simulink model "IWP_FL_ToBeChecked"  (R2022b)
settings: Solver=FixedStepAuto  StartTime=0.0  StopTime=100  RelTol=1e-3
undefined symbols (not defined in the file): a11_num, a12_num, a21_num, a22_num, g, K_aug, mc_num
settings Model: Creator=User  LastModifiedBy=User

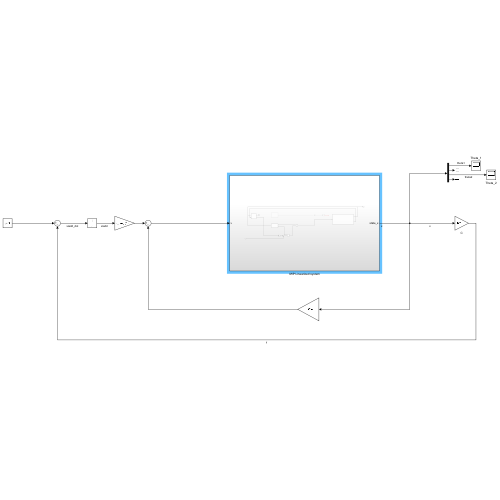
[thumbnail: Simulink's stored preview of the top-level diagram]
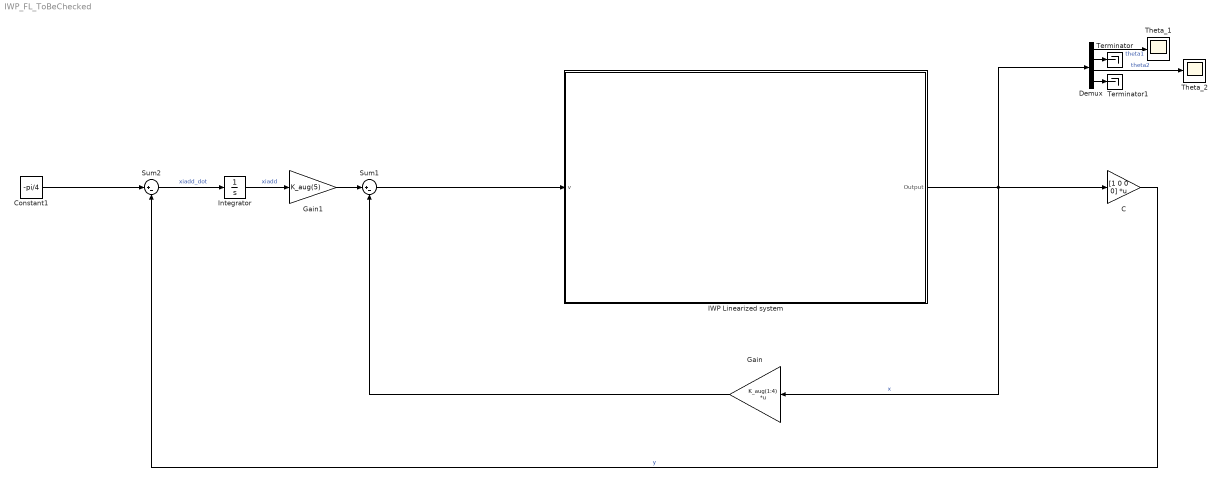
== system IWP_FL_ToBeChecked ==
  C : Gain  Gain=[1 0 0 0]  Multiplication=Matrix(K*u)
  Constant1 : Constant  Value=-pi/4
  Demux : Demux
  Gain : Gain  Gain=K_aug(1:4)  Multiplication=Matrix(K*u)  RndMeth=Simplest
  Gain1 : Gain  Gain=K_aug(5)
  IWP Linearized system : Subsystem
  Integrator : Integrator
  Sum1 : Sum  Inputs=|+-
  Sum2 : Sum  Inputs=|+-
  Terminator : Terminator
  Terminator1 : Terminator
  Theta_1 : Scope
  Theta_2 : Scope
  wires:
  Demux/2 -> Terminator/1
  Demux/4 -> Terminator1/1
  Demux/1 -> Theta_1/1  "theta1"
  Demux/3 -> Theta_2/1  "theta2"
  Gain/1 -> Sum1/2
  Sum1/1 -> IWP Linearized system/1(v)
  Gain1/1 -> Sum1/1
  Constant1/1 -> Sum2/1
  C/1 -> Sum2/2  "y"
  Sum2/1 -> Integrator/1  "xiadd_dot"
  Integrator/1 -> Gain1/1  "xiadd"
  IWP Linearized system/1(Output) -> C/1, Gain/1, Demux/1  "x"

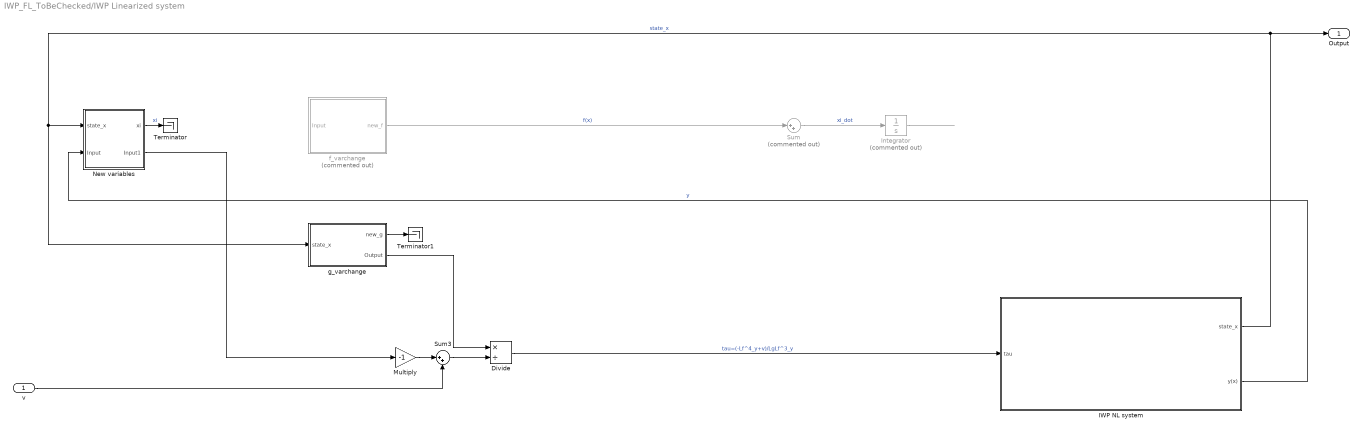
== system IWP_FL_ToBeChecked/IWP Linearized system ==
  v : Inport
  Divide : Product  Inputs=*/  RndMeth=Zero  SaturateOnIntegerOverflow=on
  IWP NL system : Subsystem
  Integrator : Integrator  Commented=on
  Multiply : Gain  Gain=-1
  New variables : Subsystem
  Sum : Sum  Commented=on  Inputs=|++
  Sum3 : Sum  Inputs=|++
  Terminator : Terminator
  Terminator1 : Terminator
  f_varchange : Subsystem  Commented=on
  g_varchange : Subsystem
  Output : Outport
  wires:
  Multiply/1 -> Sum3/1
  v/1 -> Sum3/2
  IWP NL system/1(state_x) -> g_varchange/1(state_x), New variables/1(state_x), Output/1  "state_x"
  New variables/2(Input1) -> Multiply/1
  g_varchange/2(Output) -> Divide/1
  Sum3/1 -> Divide/2
  f_varchange/1(new_f) -> Sum/1  "f(x)"
  Divide/1 -> IWP NL system/1(tau)  "tau=(-Lf^4_y+v)/LgLf^3_y"
  Sum/1 -> Integrator/1  "xi_dot"
  Integrator/1 -> ?
  IWP NL system/2(y(x)) -> New variables/2(Input)  "y"
  New variables/1(xi) -> Terminator/1  "xi"
  g_varchange/1(new_g) -> Terminator1/1

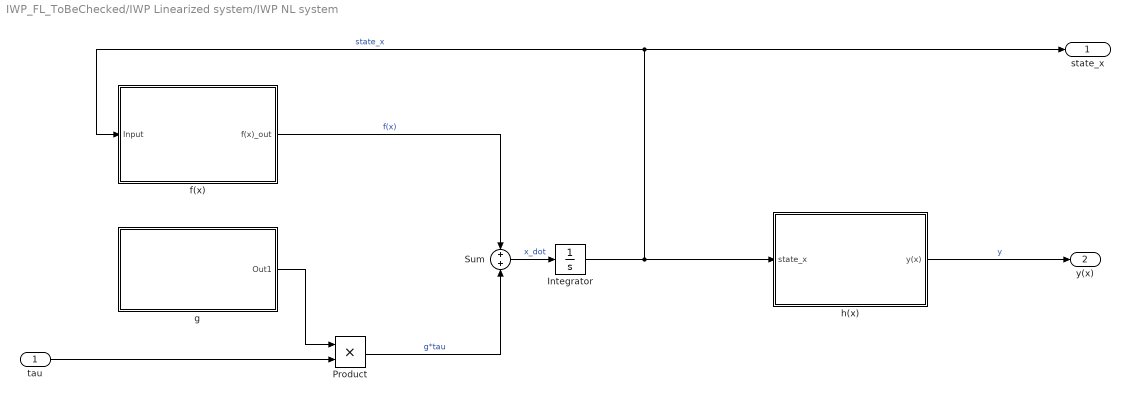
== system IWP_FL_ToBeChecked/IWP Linearized system/IWP NL system ==
  tau : Inport
  Integrator : Integrator  InitialCondition=[pi/4 0 0 0]
  Product : Product
  Sum : Sum  Inputs=+|+
  f(x) : Subsystem
  g : Subsystem
  h(x) : Subsystem
  state_x : Outport
  y(x) : Outport  Port=2
  wires:
  Product/1 -> Sum/2  "g*tau"
  Integrator/1 -> f(x)/1(Input), state_x/1, h(x)/1(state_x)  "state_x"
  g/1(Out1) -> Product/1
  f(x)/1(f(x)_out) -> Sum/1  "f(x)"
  Sum/1 -> Integrator/1  "x_dot"
  tau/1 -> Product/2
  h(x)/1(y(x)) -> y(x)/1  "y"

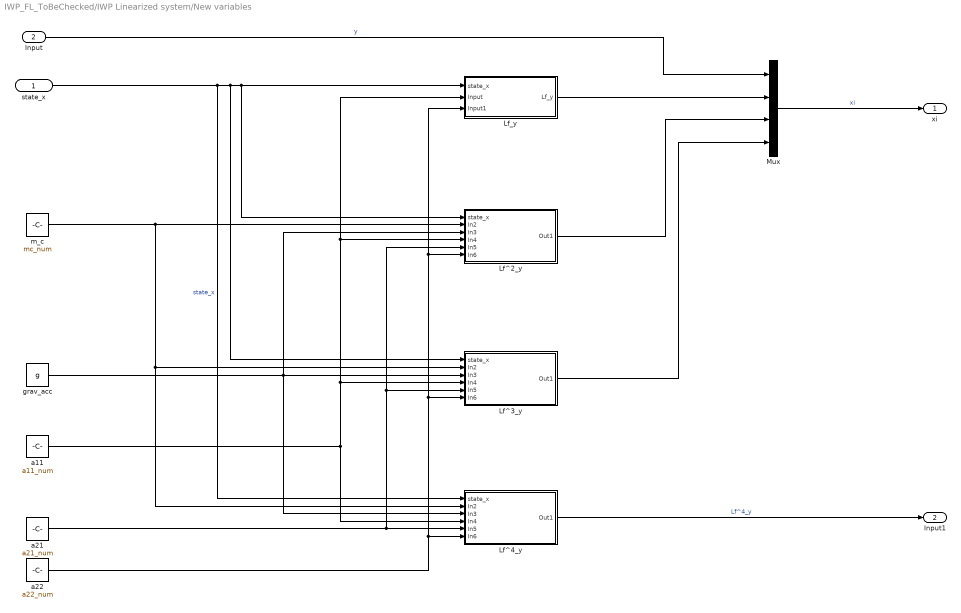
== system IWP_FL_ToBeChecked/IWP Linearized system/New variables ==
  state_x : Inport
  Input : Inport  Port=2
  Lf^2_y : Subsystem
  Lf^3_y : Subsystem
  Lf^4_y : Subsystem
  Lf_y : Subsystem
  Mux : Mux
  a11 : Constant  Value=a11_num
  a21 : Constant  Value=a21_num
  a22 : Constant  Value=a22_num
  grav_acc : Constant  Value=g
  m_c : Constant  Value=mc_num
  xi : Outport
  Input1 : Outport  Port=2
  wires:
  a22/1 -> Lf_y/3(Input1), Lf^2_y/6(In6), Lf^3_y/6(In6), Lf^4_y/6(In6)
  a11/1 -> Lf^4_y/4(In4), Lf^2_y/4(In4), Lf_y/2(Input), Lf^3_y/4(In4)
  grav_acc/1 -> Lf^2_y/3(In3), Lf^3_y/3(In3), Lf^4_y/3(In3)
  Lf^4_y/1(Out1) -> Input1/1  "Lf^4_y"
  a21/1 -> Lf^4_y/5(In5), Lf^2_y/5(In5), Lf^3_y/5(In5)
  Lf^3_y/1(Out1) -> Mux/4
  state_x/1 -> Lf^2_y/1(state_x), Lf_y/1(state_x), Lf^3_y/1(state_x), Lf^4_y/1(state_x)  "state_x"
  m_c/1 -> Lf^2_y/2(In2), Lf^3_y/2(In2), Lf^4_y/2(In2)
  Input/1 -> Mux/1  "y"
  Lf_y/1(Lf_y) -> Mux/2
  Lf^2_y/1(Out1) -> Mux/3
  Mux/1 -> xi/1  "xi"

== system IWP_FL_ToBeChecked/IWP Linearized system/f_varchange ==
  Input : Inport
  Constant : Constant  Value=0
  Demux : Demux
  Mux1 : Mux
  Terminator : Terminator
  new_f : Outport
  wires:
  Mux1/1 -> new_f/1  "new_f"
  Demux/2 -> Mux1/1
  Demux/4 -> Mux1/3
  Demux/3 -> Mux1/2
  Demux/1 -> Terminator/1
  Input/1 -> Demux/1  "xi"
  Constant/1 -> Mux1/4

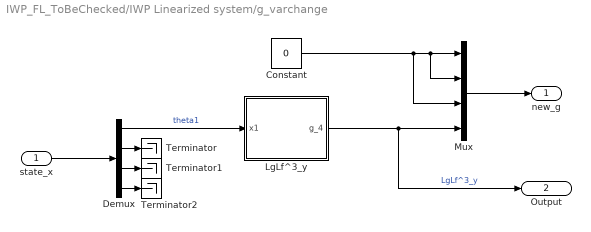
== system IWP_FL_ToBeChecked/IWP Linearized system/g_varchange ==
  state_x : Inport
  Constant : Constant  Value=0
  Demux : Demux
  LgLf^3_y : Subsystem
  Mux : Mux
  Terminator : Terminator
  Terminator1 : Terminator
  Terminator2 : Terminator
  new_g : Outport
  Output : Outport  Port=2
  wires:
  Mux/1 -> new_g/1
  Constant/1 -> Mux/3, Mux/2, Mux/1
  state_x/1 -> Demux/1
  Demux/1 -> LgLf^3_y/1(x1)  "theta1"
  LgLf^3_y/1(g_4) -> Output/1, Mux/4  "LgLf^3_y"
  Demux/2 -> Terminator/1
  Demux/3 -> Terminator1/1
  Demux/4 -> Terminator2/1

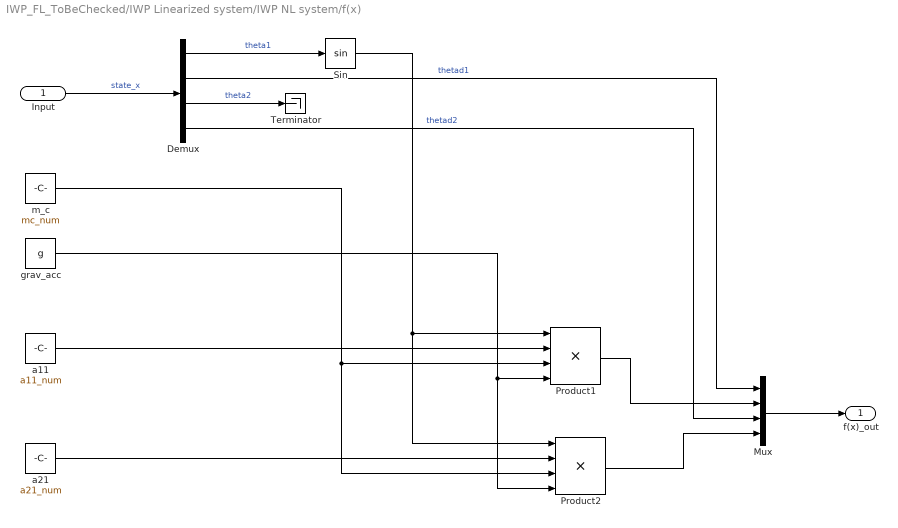
== system IWP_FL_ToBeChecked/IWP Linearized system/IWP NL system/f(x) ==
  Input : Inport
  Demux : Demux
  Mux : Mux
  Product1 : Product  Inputs=4
  Product2 : Product  Inputs=4
  Sin : Trigonometry
  Terminator : Terminator
  a11 : Constant  Value=a11_num
  a21 : Constant  Value=a21_num
  grav_acc : Constant  Value=g
  m_c : Constant  Value=mc_num
  f(x)_out : Outport
  wires:
  Demux/4 -> Mux/3  "thetad2"
  m_c/1 -> Product1/3, Product2/3
  Mux/1 -> f(x)_out/1
  grav_acc/1 -> Product1/4, Product2/4
  Product2/1 -> Mux/4
  a21/1 -> Product2/2
  a11/1 -> Product1/2
  Input/1 -> Demux/1  "state_x"
  Product1/1 -> Mux/2
  Sin/1 -> Product1/1, Product2/1
  Demux/2 -> Mux/1  "thetad1"
  Demux/1 -> Sin/1  "theta1"
  Demux/3 -> Terminator/1  "theta2"

== system IWP_FL_ToBeChecked/IWP Linearized system/IWP NL system/g ==
  Constant : Constant  Value=0
  Mux : Mux
  a12 : Constant  Value=a12_num
  a22 : Constant  Value=a22_num
  Out1 : Outport
  wires:
  a12/1 -> Mux/2
  Constant/1 -> Mux/3, Mux/1
  Mux/1 -> Out1/1  "g"
  a22/1 -> Mux/4

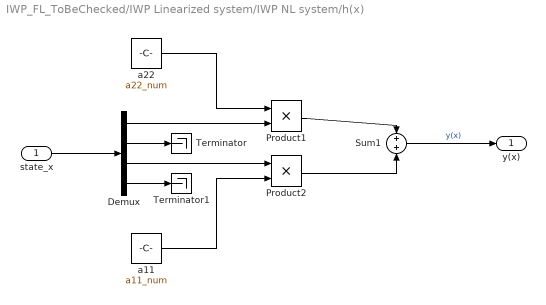
== system IWP_FL_ToBeChecked/IWP Linearized system/IWP NL system/h(x) ==
  state_x : Inport
  Demux : Demux
  Product1 : Product
  Product2 : Product
  Sum1 : Sum  Inputs=+|+
  Terminator : Terminator
  Terminator1 : Terminator
  a11 : Constant  Value=a11_num
  a22 : Constant  Value=a22_num
  y(x) : Outport
  wires:
  Demux/4 -> Terminator1/1
  Product2/1 -> Sum1/2
  Demux/1 -> Product1/2
  Demux/2 -> Terminator/1
  Demux/3 -> Product2/1
  a22/1 -> Product1/1
  state_x/1 -> Demux/1
  a11/1 -> Product2/2
  Product1/1 -> Sum1/1
  Sum1/1 -> y(x)/1  "y(x)"

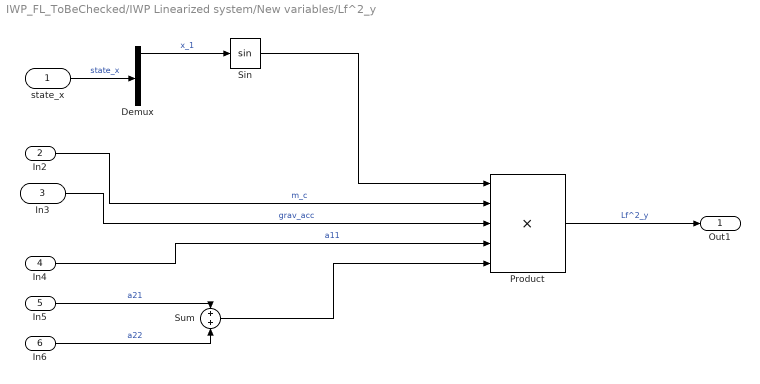
== system IWP_FL_ToBeChecked/IWP Linearized system/New variables/Lf^2_y ==
  state_x : Inport
  In2 : Inport  Port=2
  In3 : Inport  Port=3
  In4 : Inport  Port=4
  In5 : Inport  Port=5
  In6 : Inport  Port=6
  Demux : Demux
  Product : Product  Inputs=5
  Sin : Trigonometry
  Sum : Sum  Inputs=+|+
  Out1 : Outport
  wires:
  Product/1 -> Out1/1  "Lf^2_y"
  state_x/1 -> Demux/1  "state_x"
  Demux/1 -> Sin/1  "x_1"
  Sin/1 -> Product/1
  In2/1 -> Product/2  "m_c"
  In3/1 -> Product/3  "grav_acc"
  In4/1 -> Product/4  "a11"
  In5/1 -> Sum/1  "a21"
  In6/1 -> Sum/2  "a22"
  Sum/1 -> Product/5

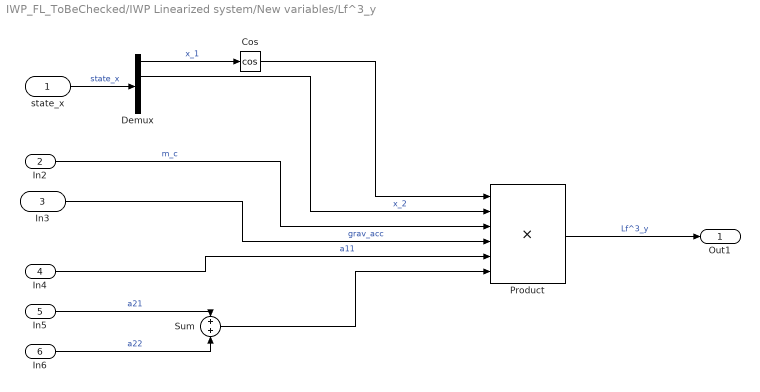
== system IWP_FL_ToBeChecked/IWP Linearized system/New variables/Lf^3_y ==
  state_x : Inport
  In2 : Inport  Port=2
  In3 : Inport  Port=3
  In4 : Inport  Port=4
  In5 : Inport  Port=5
  In6 : Inport  Port=6
  Cos : Trigonometry  Operator=cos
  Demux : Demux
  Product : Product  Inputs=6
  Sum : Sum  Inputs=+|+
  Out1 : Outport
  wires:
  Product/1 -> Out1/1  "Lf^3_y"
  state_x/1 -> Demux/1  "state_x"
  Demux/1 -> Cos/1  "x_1"
  Cos/1 -> Product/1
  In2/1 -> Product/3  "m_c"
  In3/1 -> Product/4  "grav_acc"
  In4/1 -> Product/5  "a11"
  In5/1 -> Sum/1  "a21"
  In6/1 -> Sum/2  "a22"
  Sum/1 -> Product/6
  Demux/2 -> Product/2  "x_2"

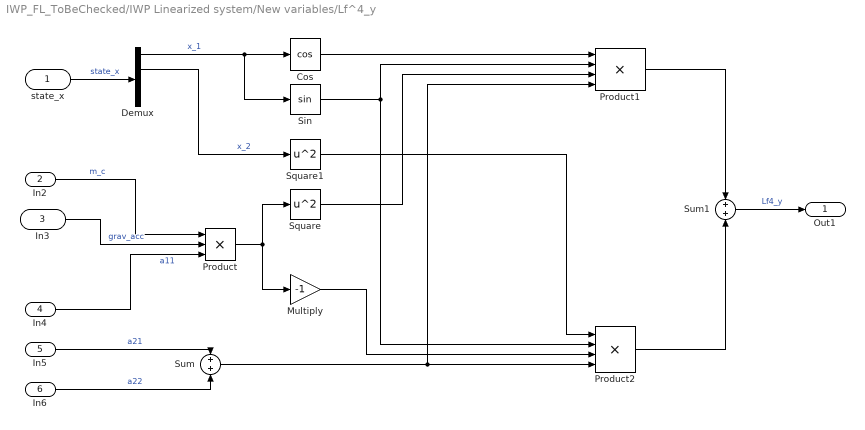
== system IWP_FL_ToBeChecked/IWP Linearized system/New variables/Lf^4_y ==
  state_x : Inport
  In2 : Inport  Port=2
  In3 : Inport  Port=3
  In4 : Inport  Port=4
  In5 : Inport  Port=5
  In6 : Inport  Port=6
  Cos : Trigonometry  Operator=cos
  Demux : Demux
  Multiply : Gain  Gain=-1
  Product : Product  Inputs=3
  Product1 : Product  Inputs=4
  Product2 : Product  Inputs=4
  Sin : Trigonometry
  Square : Math  Operator=square
  Square1 : Math  Operator=square
  Sum : Sum  Inputs=+|+
  Sum1 : Sum  Inputs=+|+
  Out1 : Outport
  wires:
  state_x/1 -> Demux/1  "state_x"
  Demux/1 -> Cos/1, Sin/1  "x_1"
  In5/1 -> Sum/1  "a21"
  In6/1 -> Sum/2  "a22"
  In2/1 -> Product/1  "m_c"
  In4/1 -> Product/3  "a11"
  In3/1 -> Product/2  "grav_acc"
  Product/1 -> Multiply/1, Square/1
  Sum1/1 -> Out1/1  "Lf4_y"
  Cos/1 -> Product1/1
  Sin/1 -> Product2/2, Product1/2
  Square/1 -> Product1/3
  Sum/1 -> Product2/4, Product1/4
  Product1/1 -> Sum1/1
  Multiply/1 -> Product2/3
  Demux/2 -> Square1/1  "x_2"
  Product2/1 -> Sum1/2
  Square1/1 -> Product2/1

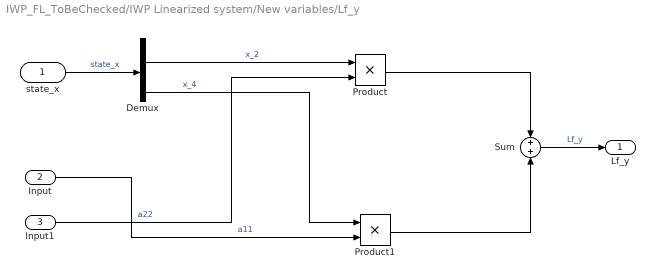
== system IWP_FL_ToBeChecked/IWP Linearized system/New variables/Lf_y ==
  state_x : Inport
  Input : Inport  Port=2
  Input1 : Inport  Port=3
  Demux : Demux
  Product : Product
  Product1 : Product
  Sum : Sum  Inputs=+|+
  Lf_y : Outport
  wires:
  state_x/1 -> Demux/1  "state_x"
  Product/1 -> Sum/1
  Product1/1 -> Sum/2
  Sum/1 -> Lf_y/1  "Lf_y"
  Demux/2 -> Product/1  "x_2"
  Demux/4 -> Product1/1  "x_4"
  Input/1 -> Product1/2  "a11"
  Input1/1 -> Product/2  "a22"

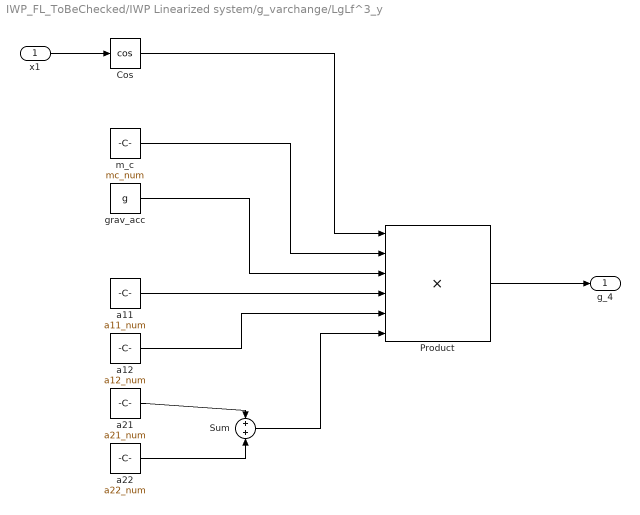
== system IWP_FL_ToBeChecked/IWP Linearized system/g_varchange/LgLf^3_y ==
  x1 : Inport
  Cos : Trigonometry  Operator=cos
  Product : Product  Inputs=6
  Sum : Sum  Inputs=+|+
  a11 : Constant  Value=a11_num
  a12 : Constant  Value=a12_num
  a21 : Constant  Value=a21_num
  a22 : Constant  Value=a22_num
  grav_acc : Constant  Value=g
  m_c : Constant  Value=mc_num
  g_4 : Outport
  wires:
  a12/1 -> Product/5
  m_c/1 -> Product/2
  a21/1 -> Sum/1
  a22/1 -> Sum/2
  a11/1 -> Product/4
  grav_acc/1 -> Product/3
  Sum/1 -> Product/6
  Cos/1 -> Product/1
  x1/1 -> Cos/1
  Product/1 -> g_4/1
